simulink model "RL_sus_quarter_sim"  (R2025a)
settings: Solver=FixedStepAuto  StartTime=0.0  StopTime=20  FixedStep=0.001  RelTol=1e-3
model workspace (MAT data in the model file):
  G0 : Simulink.Parameter (value not decoded)
  Q_F : Simulink.Parameter (value not decoded)
  Q_dot_s : Simulink.Parameter (value not decoded)
  Q_dot_s_h : Simulink.Parameter (value not decoded)
  Q_dot_u : Simulink.Parameter (value not decoded)
  Q_flec : Simulink.Parameter (value not decoded)
  Q_flec_t : Simulink.Parameter (value not decoded)
  b_deflec : Simulink.Parameter (value not decoded)
  bump_height : Simulink.Parameter (value not decoded)
  bump_lenth : Simulink.Parameter (value not decoded)
  bump_start : Simulink.Parameter (value not decoded)
  f0 : Simulink.Parameter (value not decoded)
  kt : Simulink.Parameter (value not decoded)
  ms : Simulink.Parameter (value not decoded)
  n0 : Simulink.Parameter (value not decoded)
  n1 : Simulink.Parameter (value not decoded)
  omega_1 : Simulink.Parameter (value not decoded)
  omega_2 : Simulink.Parameter (value not decoded)
  omega_3 : Simulink.Parameter (value not decoded)
  omega_4 : Simulink.Parameter (value not decoded)
  ramp_height : Simulink.Parameter (value not decoded)
  ramp_lenth : Simulink.Parameter (value not decoded)
  ramp_start : Simulink.Parameter (value not decoded)
  sine_amp : Simulink.Parameter (value not decoded)
  sine_freq : Simulink.Parameter (value not decoded)
  u : Simulink.Parameter (value not decoded)
symbols that are objects in the model workspace (value not decoded): b_deflec, bump_height, bump_lenth, bump_start, f0, G0, kt, ms, n0, n1, omega_1, omega_2, omega_3, omega_4, Q_dot_s, Q_dot_s_h, Q_F, Q_flec, Q_flec_t, ramp_height, ramp_lenth, ramp_start, sine_amp, sine_freq
undefined symbols (not defined in the file): Ground, Hook, SH_ADD_new_as_as_xdef
libraries: fl_lib x250, nesl_utility x48, sharedTrackingLibrary x34, dspstat3 x18, simulink x3, deeplib x2, slpidlib x1
(part 6 of 12)

== system RL_sus_quarter_sim/Quarter_sys/Control/Y_1/IFEKF FDC/Subsystem ==
  v_s : Inport
  v_def : Inport  Port=2
  a_s : Inport  Port=3
  Abs : Abs  SaturateOnIntegerOverflow=off
  Constant : Constant  Value=1.4*2*pi
  Constant1 : Constant  Value=1.4*2*pi
  Constant2 : Constant  Value=3
  Constant8 : Constant  Value=0
  FS2 : Constant  Value=11
  FS3 : Constant  Value=15
  MATLAB Function : MATLAB Function  TreatAsAtomicUnit=on
  MATLAB Function1 : MATLAB Function  TreatAsAtomicUnit=on
  MATLAB Function2 : Subsystem  Variant=on  VariantControlMode=label  VariantControl=MATLAB Function1  LabelModeActiveChoice=adaptive IFEKF sdimple_3
  MATLAB Function3 : MATLAB Function  TreatAsAtomicUnit=on
  Multiport Switch : MultiPortSwitch  SaturateOnIntegerOverflow=off  InputSameDT=off
  Scope : Scope
      settings: ActiveDisplayYMinimum=8.52023  ActiveDisplayYMaximum=10.23596  DataLoggingVariableName=ScopeData4
  To Workspace : ToWorkspace  VariableName=est_omega  SampleTime=-1
  Zero-Order Hold : ZeroOrderHold  SampleTime=0.001
  FS_select : Outport
  wires:
  Constant8/1 -> MATLAB Function2/2(epsilon)
  Zero-Order Hold/1 -> MATLAB Function2/1(y)
  MATLAB Function2/6(omega) -> Abs/1
  Abs/1 -> MATLAB Function/1(u), MATLAB Function3/1(u), MATLAB Function1/1(u), To Workspace/1, Scope/1
  FS2/1 -> MATLAB Function/2(FS_2), MATLAB Function1/2(FS_2), MATLAB Function3/5(alpha2)
  MATLAB Function/1(y) -> Multiport Switch/2
  v_s/1 -> MATLAB Function1/3(vs), MATLAB Function3/2(vs), MATLAB Function/3(vs), Zero-Order Hold/1
  Constant/1 -> MATLAB Function/5(alpha), MATLAB Function1/5(alpha)
  v_def/1 -> MATLAB Function/4(vdef)
  MATLAB Function1/1(y) -> Multiport Switch/3
  Multiport Switch/1 -> FS_select/1
  a_s/1 -> MATLAB Function1/4(as), MATLAB Function3/3(as)
  MATLAB Function3/1(y) -> Multiport Switch/4
  Constant2/1 -> Multiport Switch/1
  Constant1/1 -> MATLAB Function3/4(alpha)
  FS3/1 -> MATLAB Function3/6(alpha3)

== system RL_sus_quarter_sim/Quarter_sys/Control/Y_1/IFEKF FDC/Subsystem1 ==
  v_def : Inport
  Gain : Gain  Gain=-1
  Lmbada_C : Constant  Value=1000
  Product1 : Product
  Out1 : Outport
  wires:
  Gain/1 -> Out1/1
  v_def/1 -> Product1/1
  Lmbada_C/1 -> Product1/2
  Product1/1 -> Gain/1

== system RL_sus_quarter_sim/Quarter_sys/Control/Y_1/IFEKF FDC/skyhook ==
  v_def : Inport
  v_s : Inport  Port=2
  Add : Sum
  Constant : Constant  Value=-1
  Constant1 : Constant
  Delta_C : Gain  Gain=500
  Gain : Gain  Gain=-1
  Lmbada_C : Constant  Value=1000
  Product : Product
  Product1 : Product
  Switch : Switch  Criteria=u2 > Threshold  SaturateOnIntegerOverflow=off  InputSameDT=off
  F_sus1 : Outport
  wires:
  v_def/1 -> Product/1, Product1/1
  Switch/1 -> Delta_C/1
  Add/1 -> Product1/2
  Constant/1 -> Switch/3
  Lmbada_C/1 -> Add/2
  v_s/1 -> Product/2
  Delta_C/1 -> Add/1
  Constant1/1 -> Switch/1
  Product1/1 -> Gain/1
  Product/1 -> Switch/2
  Gain/1 -> F_sus1/1

== system RL_sus_quarter_sim/Quarter_sys/Control/Y_1/IFEKF SHADD/ADD ==
  v_def : Inport
  a_s : Inport  Port=2
  Add : Sum
  Constant : Constant  Value=-1
  Constant1 : Constant
  Delta_C : Gain  Gain=500
  Gain1 : Gain  Gain=-1
  Lmbada_C : Constant  Value=1000
  Product : Product
  Product2 : Product
  Switch : Switch  Criteria=u2 > Threshold  SaturateOnIntegerOverflow=off  InputSameDT=off
  Out1 : Outport
  wires:
  Gain1/1 -> Out1/1
  Product/1 -> Switch/2
  Add/1 -> Product2/2
  Switch/1 -> Delta_C/1
  a_s/1 -> Product/2
  v_def/1 -> Product/1, Product2/1
  Product2/1 -> Gain1/1
  Constant/1 -> Switch/3
  Constant1/1 -> Switch/1
  Delta_C/1 -> Add/1
  Lmbada_C/1 -> Add/2

== system RL_sus_quarter_sim/Quarter_sys/Control/Y_1/IFEKF SHADD/Subsystem ==
  v_s : Inport
  Abs : Abs  SaturateOnIntegerOverflow=off
  Constant8 : Constant  Value=0
  FS1 : Constant  Value=1.4
  FS2 : Constant  Value=11
  FS3 : Constant  Value=19
  MATLAB Function : MATLAB Function  TreatAsAtomicUnit=on
  MATLAB Function2 : Subsystem  Variant=on  VariantControlMode=label  VariantControl=MATLAB Function1  LabelModeActiveChoice=adaptive IFEKF simple
  Scope : Scope
      settings: ActiveDisplayYMinimum=-3.68957  ActiveDisplayYMaximum=33.7061  DataLoggingVariableName=ScopeData4
  Zero-Order Hold : ZeroOrderHold  SampleTime=0.001
  FS_select : Outport
  wires:
  FS3/1 -> MATLAB Function/4(FS_3)
  MATLAB Function/1(y) -> FS_select/1
  FS2/1 -> MATLAB Function/3(FS_2)
  FS1/1 -> MATLAB Function/2(FS_1)
  Abs/1 -> MATLAB Function/1(u), Scope/1
  v_s/1 -> Zero-Order Hold/1
  MATLAB Function2/6(omega) -> Abs/1
  Zero-Order Hold/1 -> MATLAB Function2/1(y)
  Constant8/1 -> MATLAB Function2/2(epsilon)

== system RL_sus_quarter_sim/Quarter_sys/Control/Y_1/IFEKF SHADD/skyhook ==
  v_def : Inport
  v_s : Inport  Port=2
  Add : Sum
  Constant : Constant  Value=-1
  Constant1 : Constant
  Delta_C : Gain  Gain=500
  Gain : Gain  Gain=-1
  Lmbada_C : Constant  Value=1000
  Product : Product
  Product1 : Product
  Switch : Switch  Criteria=u2 > Threshold  SaturateOnIntegerOverflow=off  InputSameDT=off
  F_sus1 : Outport
  wires:
  Gain/1 -> F_sus1/1
  Product/1 -> Switch/2
  Product1/1 -> Gain/1
  Constant1/1 -> Switch/1
  Delta_C/1 -> Add/1
  v_s/1 -> Product/2
  Lmbada_C/1 -> Add/2
  Constant/1 -> Switch/3
  Add/1 -> Product1/2
  Switch/1 -> Delta_C/1
  v_def/1 -> Product1/1, Product/1

== system RL_sus_quarter_sim/Quarter_sys/Control/Y_1/IFEKF Select c/Subsystem ==
  In1 : Inport
  Abs : Abs  SaturateOnIntegerOverflow=off
  Constant8 : Constant  Value=0
  FS1 : Constant  Value=1.5
  FS2 : Constant  Value=10.2
  MATLAB Function : MATLAB Function  TreatAsAtomicUnit=on
  MATLAB Function2 : Subsystem  Variant=on  VariantControlMode=label  VariantControl=MATLAB Function1  LabelModeActiveChoice=adaptive IFEKF simple
  Scope : Scope
      settings: ActiveDisplayYMinimum=-3.69078  ActiveDisplayYMaximum=33.71699  DataLoggingVariableName=ScopeData4
  To Workspace : ToWorkspace  VariableName=freq_hat  SampleTime=-1
  Zero-Order Hold : ZeroOrderHold  SampleTime=0.001
  FS_select : Outport
  wires:
  Constant8/1 -> MATLAB Function2/2(epsilon)
  MATLAB Function2/5(y_residual) -> ?
  Zero-Order Hold/1 -> MATLAB Function2/1(y)
  MATLAB Function2/6(omega) -> To Workspace/1, Abs/1
  In1/1 -> Zero-Order Hold/1
  Abs/1 -> Scope/1, MATLAB Function/1(u)
  MATLAB Function2/1(x1hat) -> ?
  MATLAB Function2/3(debug) -> ?
  MATLAB Function2/4(xhat_pred) -> ?
  MATLAB Function2/2(P) -> ?
  FS1/1 -> MATLAB Function/2(FS_1)
  FS2/1 -> MATLAB Function/3(FS_2)
  MATLAB Function/1(y) -> FS_select/1

== system RL_sus_quarter_sim/Quarter_sys/Control/Y_1/IFEKF Select c/Subsystem2 ==
  sig select : Inport
  v_def : Inport  Port=2
  v_s : Inport  Port=3
  a_s : Inport  Port=4
  constant : Subsystem  VariantControl=constant
  semi ctr : Subsystem  VariantControl=semi active ctr
  F_damper : Outport

== system RL_sus_quarter_sim/Quarter_sys/Control/Y_1/IFEKF freq b/Subsystem ==
  v_s : Inport
  Abs : Abs  SaturateOnIntegerOverflow=off
  Constant8 : Constant  Value=0
  FS1 : Constant  Value=5
  FS2 : Constant  Value=11
  FS3 : Constant  Value=19
  MATLAB Function : MATLAB Function  TreatAsAtomicUnit=on
  MATLAB Function2 : Subsystem  Variant=on  VariantControlMode=label  VariantControl=MATLAB Function1  LabelModeActiveChoice=adaptive IFEKF simple
  Scope : Scope
      settings: ActiveDisplayYMinimum=-3.69075  ActiveDisplayYMaximum=33.71678  DataLoggingVariableName=ScopeData4
  Zero-Order Hold : ZeroOrderHold  SampleTime=0.001
  FS_select : Outport
  wires:
  Constant8/1 -> MATLAB Function2/2(epsilon)
  Zero-Order Hold/1 -> MATLAB Function2/1(y)
  MATLAB Function2/6(omega) -> Abs/1
  v_s/1 -> Zero-Order Hold/1
  Abs/1 -> Scope/1, MATLAB Function/1(u)
  FS1/1 -> MATLAB Function/2(FS_1)
  FS2/1 -> MATLAB Function/3(FS_2)
  MATLAB Function/1(y) -> FS_select/1
  FS3/1 -> MATLAB Function/4(FS_3)

== system RL_sus_quarter_sim/Quarter_sys/Control/Y_1/IFEKF freq b/large b ==
  a_def : Inport
  Gain : Gain  Gain=-1
  Product1 : Product
  b : Constant  Value=30
  F_sus1 : Outport
  wires:
  a_def/1 -> Product1/1
  Product1/1 -> Gain/1
  Gain/1 -> F_sus1/1
  b/1 -> Product1/2

== system RL_sus_quarter_sim/Quarter_sys/Control/Y_1/IFEKF freq b/mid b ==
  a_def : Inport
  Gain : Gain  Gain=-1
  Product1 : Product
  b : Constant  Value=10
  Out1 : Outport
  wires:
  Product1/1 -> Gain/1
  b/1 -> Product1/2
  a_def/1 -> Product1/1
  Gain/1 -> Out1/1

== system RL_sus_quarter_sim/Quarter_sys/Control/Y_1/IFEKF freq b/small  b ==
  a_def : Inport
  Gain : Gain  Gain=-1
  Product1 : Product
  b : Constant  Value=0
  Out1 : Outport
  wires:
  Gain/1 -> Out1/1
  a_def/1 -> Product1/1
  b/1 -> Product1/2
  Product1/1 -> Gain/1

== system RL_sus_quarter_sim/Quarter_sys/Control/Y_1/IFEKF freq bc/Subsystem ==
  v_s : Inport
  Abs : Abs  SaturateOnIntegerOverflow=off
  Constant8 : Constant  Value=0
  FS1 : Constant  Value=5
  FS2 : Constant  Value=11
  FS3 : Constant  Value=19
  MATLAB Function : MATLAB Function  TreatAsAtomicUnit=on
  MATLAB Function1 : MATLAB Function  TreatAsAtomicUnit=on
  MATLAB Function2 : Subsystem  Variant=on  VariantControlMode=label  VariantControl=MATLAB Function1  LabelModeActiveChoice=adaptive IFEKF simple
  Scope : Scope
      settings: ActiveDisplayYMinimum=-3.69075  ActiveDisplayYMaximum=33.71678  DataLoggingVariableName=ScopeData4
  Scope1 : Scope
      settings: ActiveDisplayYMinimum=0.875  ActiveDisplayYMaximum=2.125  DataLoggingVariableName=ScopeData9
  Scope2 : Scope
      settings: ActiveDisplayYMinimum=0.75  ActiveDisplayYMaximum=3.25  DataLoggingVariableName=ScopeData10
  Zero-Order Hold : ZeroOrderHold  SampleTime=0.001
  c FS1 : Constant  Value=1.5
  c FS2 : Constant  Value=11
  FS_select b : Outport
  FS_select c : Outport  Port=2
  wires:
  FS3/1 -> MATLAB Function/4(FS_3)
  MATLAB Function/1(y) -> Scope2/1, FS_select b/1
  FS2/1 -> MATLAB Function/3(FS_2)
  FS1/1 -> MATLAB Function/2(FS_1)
  Abs/1 -> MATLAB Function/1(u), Scope/1, MATLAB Function1/1(u)
  v_s/1 -> Zero-Order Hold/1
  MATLAB Function2/6(omega) -> Abs/1
  Zero-Order Hold/1 -> MATLAB Function2/1(y)
  Constant8/1 -> MATLAB Function2/2(epsilon)
  MATLAB Function1/1(y) -> Scope1/1, FS_select c/1
  c FS1/1 -> MATLAB Function1/2(FS_1)
  c FS2/1 -> MATLAB Function1/3(FS_2)

== system RL_sus_quarter_sim/Quarter_sys/Control/Y_1/IFEKF freq bc/large C ==
  v_def : Inport
  C : Constant  Value=2000
  Gain : Gain  Gain=-1
  Product1 : Product
  F_sus1 : Outport
  wires:
  v_def/1 -> Product1/1
  Product1/1 -> Gain/1
  Gain/1 -> F_sus1/1
  C/1 -> Product1/2

== system RL_sus_quarter_sim/Quarter_sys/Control/Y_1/IFEKF freq bc/large b ==
  a_def : Inport
  Gain : Gain  Gain=-1
  Product1 : Product
  b : Constant  Value=30
  F_sus1 : Outport
  wires:
  b/1 -> Product1/2
  Gain/1 -> F_sus1/1
  Product1/1 -> Gain/1
  a_def/1 -> Product1/1

== system RL_sus_quarter_sim/Quarter_sys/Control/Y_1/IFEKF freq bc/mid b ==
  a_def : Inport
  Gain : Gain  Gain=-1
  Product1 : Product
  b : Constant  Value=10
  Out1 : Outport
  wires:
  Gain/1 -> Out1/1
  a_def/1 -> Product1/1
  b/1 -> Product1/2
  Product1/1 -> Gain/1

== system RL_sus_quarter_sim/Quarter_sys/Control/Y_1/IFEKF freq bc/small  b ==
  a_def : Inport
  Gain : Gain  Gain=-1
  Product1 : Product
  b : Constant  Value=0
  Out1 : Outport
  wires:
  Product1/1 -> Gain/1
  b/1 -> Product1/2
  a_def/1 -> Product1/1
  Gain/1 -> Out1/1

== system RL_sus_quarter_sim/Quarter_sys/Control/Y_1/IFEKF freq bc/small C ==
  v_def : Inport
  C : Constant  Value=1000
  Gain : Gain  Gain=-1
  Product1 : Product
  Out1 : Outport
  wires:
  Gain/1 -> Out1/1
  v_def/1 -> Product1/1
  C/1 -> Product1/2
  Product1/1 -> Gain/1

== system RL_sus_quarter_sim/Quarter_sys/Control/Y_1/IFEKF freq bkkcc/Subsystem ==
  v_s : Inport
  Abs : Abs  SaturateOnIntegerOverflow=off
  Chart : Stateflow chart  TreatAsAtomicUnit=on  SystemSampleTime=0.001
  Chart1 : Stateflow chart  TreatAsAtomicUnit=on  SystemSampleTime=0.001
  Constant : Constant  Value=10000
  Constant1 : Constant  Value=10
  Constant2 : Constant  Value=1000
  Constant3 : Constant  Value=-500
  Constant4 : Constant  Value=-10000
  Constant5 : Constant  Value=30
  Constant6 : Constant  Value=3
  Constant8 : Constant  Value=0
  Demux : Demux  Outputs=2
  FS1 : Constant  Value=0.65
  FS2 : Constant  Value=4.5
  L1 : Subsystem
  L2 : Subsystem
  L3 : Subsystem
  MATLAB Function2 : Subsystem  Variant=on  VariantControlMode=label  VariantControl=MATLAB Function1  LabelModeActiveChoice=adaptive IFEKF simple
  Manual Switch : ManualSwitch
  Multiport Switch : MultiPortSwitch  Inputs=2  SaturateOnIntegerOverflow=off  InputSameDT=off
  Multiport Switch1 : MultiPortSwitch  Inputs=7  SaturateOnIntegerOverflow=off  InputSameDT=off
  Mux : Mux
  Mux1 : Mux  Inputs=2
  Mux2 : Mux  Inputs=2
  Scope : Scope
      settings: ActiveDisplayYMinimum=7.5  ActiveDisplayYMaximum=32.5
  Scope1 : Scope
      settings: ActiveDisplayYMinimum=-10696.7424  ActiveDisplayYMaximum=10249.86115  DataLoggingVariableName=ScopeData2
  Scope2 : Scope
      settings: ActiveDisplayYMinimum=0.875  ActiveDisplayYMaximum=2.125  DataLoggingVariableName=ScopeData3
  Zero-Order Hold : ZeroOrderHold  SampleTime=0.001
  passive : Subsystem
  Out1 : Outport
  wires:
  Constant8/1 -> MATLAB Function2/2(epsilon)
  Zero-Order Hold/1 -> MATLAB Function2/1(y)
  MATLAB Function2/6(omega) -> Abs/1
  v_s/1 -> Zero-Order Hold/1
  Abs/1 -> Chart/1(freq), Chart1/1(freq)
  FS1/1 -> Chart/2(FS1)
  FS2/1 -> Chart/3(FS2)
  Demux/1 -> Mux/1, Scope1/1  "k_a1"
  Constant3/1 -> Mux/2  "c_a1"
  Constant2/1 -> Mux/3  "c_a2"
  Demux/2 -> Scope/1, Mux/4  "b"
  Mux/1 -> ?
  Chart/1(level) -> Multiport Switch/1
  Multiport Switch/1 -> Demux/1
  Constant/1 -> Mux1/1  "ka1"
  Constant1/1 -> Mux1/2  "b"
  Mux1/1 -> Multiport Switch/2  "L1"
  Constant4/1 -> Mux2/1  "ka1"
  Constant5/1 -> Mux2/2  "b"
  Mux2/1 -> Multiport Switch/3  "L2"
  Chart1/1(level) -> Scope2/1, Manual Switch/1
  Multiport Switch1/1 -> Out1/1
  L1/1(Out1) -> Multiport Switch1/5, Multiport Switch1/8
  Manual Switch/1 -> Multiport Switch1/1
  Constant6/1 -> Manual Switch/2
  L3/1(Out1) -> Multiport Switch1/4, Multiport Switch1/7
  L2/1(Out1) -> Multiport Switch1/2, Multiport Switch1/3
  passive/1(Out1) -> Multiport Switch1/6

== system RL_sus_quarter_sim/Quarter_sys/Control/Y_1/IFEKF freq bkkcc/Subsystem1 ==
  input1 : Inport
  input0 : Inport  Port=2
  Ideal Force Sensor : fl_lib/Mechanical/Mechanical Sensors/Ideal Force Sensor
  Ideal Translational Velocity Source : fl_lib/Mechanical/Mechanical Sources/Ideal Translational Velocity Source
  Mechanical Translational Reference : fl_lib/Mechanical/Translational Elements/Mechanical Translational Reference
  Mechanical Translational Reference1 : fl_lib/Mechanical/Translational Elements/Mechanical Translational Reference
  PS-Simulink Converter : nesl_utility/PS-Simulink Converter  PhysicalDomain=network_engine_domain  SubClassName=ps_output  LeftPortType=input  RightPortType=output  PseudoPeriodic=off  Frequencies=[]  VectorFormat=inherit  Unit=inherit  AffineConversion=off
  Simulink-PS Converter : nesl_utility/Simulink-PS Converter  PhysicalDomain=network_engine_domain  SubClassName=ps_input  LeftPortType=input  RightPortType=output  PseudoPeriodic=off  Frequencies=[]  NoiseDistribution=none  NoiseParameters=[]  Unit=1  AffineConversion=off  FilteringAndDerivatives=provide  SimscapeFilterOrder=1  InputFilterTimeConstant=0.001  UdotUserProvided=1
  Solver Configuration : nesl_utility/Solver Configuration  PhysicalDomain=network_engine_domain  SubClassName=solver  LeftPortType=input  RightPortType=generic  Tones=[]  Harmonics=[]  SimulateNoise=off  Profile=off  UseLocalSampling=off  EnableSwitchedLinearOptims=on  FrequencyDomain=off  UseCCode=off  RelTol=0.001  AbsTol=0.001  MinStep=1e-09  ToWorkspace=off  RevertToSquareIcSolve=off  NumHomotopyIterations=100  PhasorMode=off  PhasorModeNumHarmonics=1  ConsistencySolver=NEWTON_XTOL_AFTER_FTOL  IndexReductionMethod=DerivativeReplacement  DoDC=off  ResidualTolerance=1e-09  ConsistencyTolSource=GLOBAL  ConsistencyAbsTol=0.001  ConsistencyRelTol=0.001  ConsistencyTolFactor=0.001  UseLocalSolver=off  LocalSolverChoice=NE_BACKWARD_EULER_ADVANCER  ResolveIndetEquations=on  FunctionEvalNumThread=1  LocalSolverSampleTime=0.001  DoFixedCost=off  MaxNonlinIter=3  MaxModeIter=2  ComputeImpulses=off  ImpulseIterations=2  LinearAlgebra=auto  LinearAlgebraNumThread=0  EquationFormulation=NE_TIME_EF  DelaysMemoryBudget=1024  AutomaticFiltering=on  FilteringTimeConstant=0.001  PartitionStorageMethod=AS_NEEDED  PartitionMemoryBudget=1024  PartitionMethod=ROBUST  MultibodyUseLocalSolver=off  MultibodyLocalSolverChoice=ODE1  MultibodyLocalSolverSampleTime=0.001
  Subsystem1 : Subsystem
  output : Outport
  wires:
  PS-Simulink Converter/1 -> output/1
  input0/1 -> Simulink-PS Converter/1
  input1/1 -> Simulink-PS Converter/2
  connections:
  Simulink-PS Converter/RConn1 -- Ideal Translational Velocity Source/RConn1
  Subsystem1/LConn1 -- Ideal Translational Velocity Source/RConn2
  Ideal Force Sensor/RConn1 -- Mechanical Translational Reference/LConn1
  Ideal Force Sensor/LConn1 -- Subsystem1/RConn1
  Mechanical Translational Reference1/LConn1 -- Solver Configuration/RConn1 -- Ideal Translational Velocity Source/LConn1
  PS-Simulink Converter/LConn1 -- Ideal Force Sensor/RConn2

== system RL_sus_quarter_sim/Quarter_sys/Control/Y_1/IFEKF freq bkkcc/bkkcc ==
  v_def : Inport
  x_def : Inport  Port=2
  a_def : Inport  Port=3
  param_ctr : Inport  Port=4
  Add : Sum  Inputs=+++
  Add1 : Sum
  Demux : Demux
  Divide : Product  Inputs=*/
  Gain{,1..3} (4 alike) : Gain  Gain=-1
  Integrator : Integrator
  Product{,1..3} (4 alike) : Product
  F_bkkcc : Outport
  wires:
  x_def/1 -> Product/2
  Demux/1 -> Gain/1  "k_a1"
  Product/1 -> Add/1
  Demux/2 -> Gain1/1  "c_a1"
  Product1/1 -> Add/2
  Add/1 -> F_bkkcc/1
  Demux/3 -> Product3/1, Gain2/1  "c_a2"
  Demux/4 -> Gain3/1  "b"
  Product2/1 -> Add/3
  Gain/1 -> Product/1
  Gain1/1 -> Product1/1
  Gain2/1 -> Product2/1
  Gain3/1 -> Divide/2
  param_ctr/1 -> Demux/1
  Add1/1 -> Integrator/1  "a1"
  Divide/1 -> Add1/1
  a_def/1 -> Add1/2
  v_def/1 -> Product1/2
  Integrator/1 -> Product2/2, Product3/2  "v1"
  Product3/1 -> Divide/1

== system RL_sus_quarter_sim/Quarter_sys/Control/Y_1/IFEKF freq c/Large C ==
  v_def : Inport
  Gain : Gain  Gain=-1
  Lmbada_C : Constant  Value=1500
  Product1 : Product
  Out1 : Outport
  wires:
  Gain/1 -> Out1/1
  v_def/1 -> Product1/1
  Lmbada_C/1 -> Product1/2
  Product1/1 -> Gain/1

== system RL_sus_quarter_sim/Quarter_sys/Control/Y_1/IFEKF freq c/Mid C ==
  v_def : Inport
  Gain : Gain  Gain=-1
  Lmbada_C : Constant  Value=1000
  Product1 : Product
  Out1 : Outport
  wires:
  Gain/1 -> Out1/1
  v_def/1 -> Product1/1
  Lmbada_C/1 -> Product1/2
  Product1/1 -> Gain/1

== system RL_sus_quarter_sim/Quarter_sys/Control/Y_1/IFEKF freq c/Small C ==
  v_def : Inport
  Gain : Gain  Gain=-1
  Lmbada_C : Constant  Value=500
  Product1 : Product
  Out1 : Outport
  wires:
  Product1/1 -> Gain/1
  Lmbada_C/1 -> Product1/2
  v_def/1 -> Product1/1
  Gain/1 -> Out1/1

== system RL_sus_quarter_sim/Quarter_sys/Control/Y_1/IFEKF freq c/Subsystem ==
  v_s : Inport
  Abs : Abs  SaturateOnIntegerOverflow=off
  Constant8 : Constant  Value=0
  FF-1 : Constant  Value=11.3
  FL-1 : Constant  Value=1.33
  FL-2 : Constant  Value=12.4
  MATLAB Function : MATLAB Function  TreatAsAtomicUnit=on
  MATLAB Function2 : Subsystem  Variant=on  VariantControlMode=label  VariantControl=MATLAB Function1  LabelModeActiveChoice=adaptive IFEKF simple
  Scope : Scope
      settings: ActiveDisplayYMinimum=-0.50296  ActiveDisplayYMaximum=5.02664  DataLoggingVariableName=ScopeData4
  Zero-Order Hold : ZeroOrderHold  SampleTime=0.001
  FS_select : Outport
  wires:
  Constant8/1 -> MATLAB Function2/2(epsilon)
  Zero-Order Hold/1 -> MATLAB Function2/1(y)
  MATLAB Function2/6(omega) -> Abs/1
  v_s/1 -> Zero-Order Hold/1
  Abs/1 -> Scope/1, MATLAB Function/1(u)
  FL-1/1 -> MATLAB Function/2(FS_1)
  FF-1/1 -> MATLAB Function/3(FS_2)
  MATLAB Function/1(y) -> FS_select/1
  FL-2/1 -> MATLAB Function/4(FS_3)

== system RL_sus_quarter_sim/Quarter_sys/Control/Y_1/PA bk/Subsystem ==
  input0 : Inport
  input1 : Inport  Port=2
  Ideal Force Sensor : fl_lib/Mechanical/Mechanical Sensors/Ideal Force Sensor
  Ideal Translational Velocity Source : fl_lib/Mechanical/Mechanical Sources/Ideal Translational Velocity Source
  Mechanical Translational Reference : fl_lib/Mechanical/Translational Elements/Mechanical Translational Reference
  Mechanical Translational Reference1 : fl_lib/Mechanical/Translational Elements/Mechanical Translational Reference
  PS-Simulink Converter : nesl_utility/PS-Simulink Converter  PhysicalDomain=network_engine_domain  SubClassName=ps_output  LeftPortType=input  RightPortType=output  PseudoPeriodic=off  Frequencies=[]  VectorFormat=inherit  Unit=inherit  AffineConversion=off
  Simulink-PS Converter : nesl_utility/Simulink-PS Converter  PhysicalDomain=network_engine_domain  SubClassName=ps_input  LeftPortType=input  RightPortType=output  PseudoPeriodic=off  Frequencies=[]  NoiseDistribution=none  NoiseParameters=[]  Unit=1  AffineConversion=off  FilteringAndDerivatives=provide  SimscapeFilterOrder=1  InputFilterTimeConstant=0.001  UdotUserProvided=1
  Solver Configuration : nesl_utility/Solver Configuration  PhysicalDomain=network_engine_domain  SubClassName=solver  LeftPortType=input  RightPortType=generic  Tones=[]  Harmonics=[]  SimulateNoise=off  Profile=off  UseLocalSampling=off  EnableSwitchedLinearOptims=on  FrequencyDomain=off  UseCCode=off  RelTol=0.001  AbsTol=0.001  MinStep=1e-09  ToWorkspace=off  RevertToSquareIcSolve=off  NumHomotopyIterations=100  PhasorMode=off  PhasorModeNumHarmonics=1  ConsistencySolver=NEWTON_XTOL_AFTER_FTOL  IndexReductionMethod=DerivativeReplacement  DoDC=off  ResidualTolerance=1e-09  ConsistencyTolSource=GLOBAL  ConsistencyAbsTol=0.001  ConsistencyRelTol=0.001  ConsistencyTolFactor=0.001  UseLocalSolver=off  LocalSolverChoice=NE_BACKWARD_EULER_ADVANCER  ResolveIndetEquations=on  FunctionEvalNumThread=1  LocalSolverSampleTime=0.001  DoFixedCost=off  MaxNonlinIter=3  MaxModeIter=2  ComputeImpulses=off  ImpulseIterations=2  LinearAlgebra=auto  LinearAlgebraNumThread=0  EquationFormulation=NE_TIME_EF  DelaysMemoryBudget=1024  AutomaticFiltering=on  FilteringTimeConstant=0.001  PartitionStorageMethod=AS_NEEDED  PartitionMemoryBudget=1024  PartitionMethod=ROBUST  MultibodyUseLocalSolver=off  MultibodyLocalSolverChoice=ODE1  MultibodyLocalSolverSampleTime=0.001
  Subsystem1 : Subsystem
  output : Outport
  wires:
  PS-Simulink Converter/1 -> output/1
  input0/1 -> Simulink-PS Converter/1
  input1/1 -> Simulink-PS Converter/2
  connections:
  Simulink-PS Converter/RConn1 -- Ideal Translational Velocity Source/RConn1
  Subsystem1/LConn1 -- Ideal Translational Velocity Source/RConn2
  Ideal Force Sensor/RConn1 -- Mechanical Translational Reference/LConn1
  Ideal Force Sensor/LConn1 -- Subsystem1/RConn1
  Solver Configuration/RConn1 -- Ideal Translational Velocity Source/LConn1 -- Mechanical Translational Reference1/LConn1
  PS-Simulink Converter/LConn1 -- Ideal Force Sensor/RConn2

== system RL_sus_quarter_sim/Quarter_sys/Control/Y_1/PA bkc/Subsystem ==
  input0 : Inport
  input1 : Inport  Port=2
  Ideal Force Sensor : fl_lib/Mechanical/Mechanical Sensors/Ideal Force Sensor
  Ideal Translational Velocity Source : fl_lib/Mechanical/Mechanical Sources/Ideal Translational Velocity Source
  Mechanical Translational Reference : fl_lib/Mechanical/Translational Elements/Mechanical Translational Reference
  Mechanical Translational Reference1 : fl_lib/Mechanical/Translational Elements/Mechanical Translational Reference
  PS-Simulink Converter : nesl_utility/PS-Simulink Converter  PhysicalDomain=network_engine_domain  SubClassName=ps_output  LeftPortType=input  RightPortType=output  PseudoPeriodic=off  Frequencies=[]  VectorFormat=inherit  Unit=inherit  AffineConversion=off
  Simulink-PS Converter : nesl_utility/Simulink-PS Converter  PhysicalDomain=network_engine_domain  SubClassName=ps_input  LeftPortType=input  RightPortType=output  PseudoPeriodic=off  Frequencies=[]  NoiseDistribution=none  NoiseParameters=[]  Unit=1  AffineConversion=off  FilteringAndDerivatives=provide  SimscapeFilterOrder=1  InputFilterTimeConstant=0.001  UdotUserProvided=1
  Solver Configuration : nesl_utility/Solver Configuration  PhysicalDomain=network_engine_domain  SubClassName=solver  LeftPortType=input  RightPortType=generic  Tones=[]  Harmonics=[]  SimulateNoise=off  Profile=off  UseLocalSampling=off  EnableSwitchedLinearOptims=on  FrequencyDomain=off  UseCCode=off  RelTol=0.001  AbsTol=0.001  MinStep=1e-09  ToWorkspace=off  RevertToSquareIcSolve=off  NumHomotopyIterations=100  PhasorMode=off  PhasorModeNumHarmonics=1  ConsistencySolver=NEWTON_XTOL_AFTER_FTOL  IndexReductionMethod=DerivativeReplacement  DoDC=off  ResidualTolerance=1e-09  ConsistencyTolSource=GLOBAL  ConsistencyAbsTol=0.001  ConsistencyRelTol=0.001  ConsistencyTolFactor=0.001  UseLocalSolver=off  LocalSolverChoice=NE_BACKWARD_EULER_ADVANCER  ResolveIndetEquations=on  FunctionEvalNumThread=1  LocalSolverSampleTime=0.001  DoFixedCost=off  MaxNonlinIter=3  MaxModeIter=2  ComputeImpulses=off  ImpulseIterations=2  LinearAlgebra=auto  LinearAlgebraNumThread=0  EquationFormulation=NE_TIME_EF  DelaysMemoryBudget=1024  AutomaticFiltering=on  FilteringTimeConstant=0.001  PartitionStorageMethod=AS_NEEDED  PartitionMemoryBudget=1024  PartitionMethod=ROBUST  MultibodyUseLocalSolver=off  MultibodyLocalSolverChoice=ODE1  MultibodyLocalSolverSampleTime=0.001
  Subsystem1 : Subsystem
  output : Outport
  wires:
  input1/1 -> Simulink-PS Converter/2
  input0/1 -> Simulink-PS Converter/1
  PS-Simulink Converter/1 -> output/1
  connections:
  PS-Simulink Converter/LConn1 -- Ideal Force Sensor/RConn2
  Ideal Translational Velocity Source/LConn1 -- Solver Configuration/RConn1 -- Mechanical Translational Reference1/LConn1
  Ideal Force Sensor/LConn1 -- Subsystem1/RConn1
  Ideal Force Sensor/RConn1 -- Mechanical Translational Reference/LConn1
  Subsystem1/LConn1 -- Ideal Translational Velocity Source/RConn2
  Simulink-PS Converter/RConn1 -- Ideal Translational Velocity Source/RConn1

== system RL_sus_quarter_sim/Quarter_sys/Control/Y_1/PA bkkcc/Subsystem ==
  input0 : Inport
  input1 : Inport  Port=2
  Ideal Force Sensor : fl_lib/Mechanical/Mechanical Sensors/Ideal Force Sensor
  Ideal Translational Velocity Source : fl_lib/Mechanical/Mechanical Sources/Ideal Translational Velocity Source
  Mechanical Translational Reference : fl_lib/Mechanical/Translational Elements/Mechanical Translational Reference
  Mechanical Translational Reference1 : fl_lib/Mechanical/Translational Elements/Mechanical Translational Reference
  PS-Simulink Converter : nesl_utility/PS-Simulink Converter  PhysicalDomain=network_engine_domain  SubClassName=ps_output  LeftPortType=input  RightPortType=output  PseudoPeriodic=off  Frequencies=[]  VectorFormat=inherit  Unit=inherit  AffineConversion=off
  Simulink-PS Converter : nesl_utility/Simulink-PS Converter  PhysicalDomain=network_engine_domain  SubClassName=ps_input  LeftPortType=input  RightPortType=output  PseudoPeriodic=off  Frequencies=[]  NoiseDistribution=none  NoiseParameters=[]  Unit=1  AffineConversion=off  FilteringAndDerivatives=provide  SimscapeFilterOrder=1  InputFilterTimeConstant=0.001  UdotUserProvided=1
  Solver Configuration : nesl_utility/Solver Configuration  PhysicalDomain=network_engine_domain  SubClassName=solver  LeftPortType=input  RightPortType=generic  Tones=[]  Harmonics=[]  SimulateNoise=off  Profile=off  UseLocalSampling=off  EnableSwitchedLinearOptims=on  FrequencyDomain=off  UseCCode=off  RelTol=0.001  AbsTol=0.001  MinStep=1e-09  ToWorkspace=off  RevertToSquareIcSolve=off  NumHomotopyIterations=100  PhasorMode=off  PhasorModeNumHarmonics=1  ConsistencySolver=NEWTON_XTOL_AFTER_FTOL  IndexReductionMethod=DerivativeReplacement  DoDC=off  ResidualTolerance=1e-09  ConsistencyTolSource=GLOBAL  ConsistencyAbsTol=0.001  ConsistencyRelTol=0.001  ConsistencyTolFactor=0.001  UseLocalSolver=off  LocalSolverChoice=NE_BACKWARD_EULER_ADVANCER  ResolveIndetEquations=on  FunctionEvalNumThread=1  LocalSolverSampleTime=0.001  DoFixedCost=off  MaxNonlinIter=3  MaxModeIter=2  ComputeImpulses=off  ImpulseIterations=2  LinearAlgebra=auto  LinearAlgebraNumThread=0  EquationFormulation=NE_TIME_EF  DelaysMemoryBudget=1024  AutomaticFiltering=on  FilteringTimeConstant=0.001  PartitionStorageMethod=AS_NEEDED  PartitionMemoryBudget=1024  PartitionMethod=ROBUST  MultibodyUseLocalSolver=off  MultibodyLocalSolverChoice=ODE1  MultibodyLocalSolverSampleTime=0.001
  Subsystem1 : Subsystem
  output : Outport
  wires:
  PS-Simulink Converter/1 -> output/1
  input0/1 -> Simulink-PS Converter/1
  input1/1 -> Simulink-PS Converter/2
  connections:
  Simulink-PS Converter/RConn1 -- Ideal Translational Velocity Source/RConn1
  Subsystem1/LConn1 -- Ideal Translational Velocity Source/RConn2
  Ideal Force Sensor/RConn1 -- Mechanical Translational Reference/LConn1
  Ideal Force Sensor/LConn1 -- Subsystem1/RConn1
  Mechanical Translational Reference1/LConn1 -- Solver Configuration/RConn1 -- Ideal Translational Velocity Source/LConn1
  PS-Simulink Converter/LConn1 -- Ideal Force Sensor/RConn2

== system RL_sus_quarter_sim/Quarter_sys/Control/Y_1/P_0/Subsystem ==
  p0_k2 : Subsystem  VariantControl=p0_k2
  p0_k3 : Subsystem  VariantControl=p0_k3
  p0_k4 : Subsystem  VariantControl=p0_k4
  p0_k6 : Subsystem  VariantControl=p0_k6
  passive : Subsystem  VariantControl=passive
  Conn1 : PMIOPort  Side=Right
  Conn2 : PMIOPort  Port=2  Side=Left

== system RL_sus_quarter_sim/Quarter_sys/Control/Y_1/P_1/Subsystem ==
  p1_k1 : Subsystem  VariantControl=p1_k1
  p1_k2 : Subsystem  VariantControl=p1_k2
  p1_k3 : Subsystem  VariantControl=p1_k3
  p1_k5 : Subsystem  VariantControl=p1_k5
  passive : Subsystem  VariantControl=passive
  Conn1 : PMIOPort  Side=Right
  Conn2 : PMIOPort  Port=2  Side=Left

== system RL_sus_quarter_sim/Quarter_sys/Control/Y_1/P_test/Subsystem ==
  p1_k1 : Subsystem  VariantControl=p1_k1
  p1_k2 : Subsystem  VariantControl=p1_k2
  p1_k3 : Subsystem  VariantControl=p1_k3
  p1_k5 : Subsystem  VariantControl=p1_k5
  passive : Subsystem  VariantControl=passive
  Conn1 : PMIOPort  Side=Right
  Conn2 : PMIOPort  Port=2  Side=Left

== system RL_sus_quarter_sim/Quarter_sys/Control/Y_1/Pabbkk/Subsystem ==
  p1_k1 : Subsystem  VariantControl=p1_k1
  p1_k2 : Subsystem  VariantControl=p1_k2
  p1_k3 : Subsystem  VariantControl=p1_k3
  p1_k5 : Subsystem  VariantControl=p1_k5
  passive : Subsystem  VariantControl=passive
  Conn1 : PMIOPort  Side=Right
  Conn2 : PMIOPort  Port=2  Side=Left

== system RL_sus_quarter_sim/Quarter_sys/Control/Y_1/SH_ADD_modify/ADD1 ==
  v_def : Inport
  a_s : Inport  Port=2
  Constant2 : Constant  Value=500
  Constant3 : Constant  Value=1500
  Product : Product
  Switch : Switch  Criteria=u2 > Threshold  SaturateOnIntegerOverflow=off  InputSameDT=off
  F_sus1 : Outport
  wires:
  Product/1 -> Switch/2
  Constant2/1 -> Switch/3
  a_s/1 -> Product/2
  v_def/1 -> Product/1
  Constant3/1 -> Switch/1
  Switch/1 -> F_sus1/1

== system RL_sus_quarter_sim/Quarter_sys/Control/Y_1/SH_ADD_modify/Modify_SHADD ==
  v_def : Inport
  a_s : Inport  Port=2
  v_s : Inport  Port=3
  Multiport Switch1 : MultiPortSwitch  Inputs=2  SaturateOnIntegerOverflow=off  InputSameDT=off
  currency_ctr1 : Outport
  wires:
  Multiport Switch1/1 -> currency_ctr1/1

== system RL_sus_quarter_sim/Quarter_sys/Control/Y_1/SH_ADD_modify/SH1 ==
  v_def : Inport
  v_s : Inport  Port=2
  Constant2 : Constant  Value=500
  Constant3 : Constant  Value=1500
  Product : Product
  Switch : Switch  Criteria=u2 > Threshold  SaturateOnIntegerOverflow=off  InputSameDT=off
  Out1 : Outport
  wires:
  Product/1 -> Switch/2
  Constant3/1 -> Switch/1
  Constant2/1 -> Switch/3
  v_def/1 -> Product/1
  v_s/1 -> Product/2
  Switch/1 -> Out1/1

== system RL_sus_quarter_sim/Quarter_sys/Control/Y_1/SH_ADD_new_FS/Modify_SHADD ==
  v_def : Inport
  a_s : Inport  Port=2
  v_s : Inport  Port=3
  ADD1 : Subsystem
  Gain1 : Gain  Gain=2*pi
  MATLAB Function : MATLAB Function  TreatAsAtomicUnit=on
  Multiport Switch1 : MultiPortSwitch  Inputs=2  SaturateOnIntegerOverflow=off  InputSameDT=off
  SH1 : Subsystem
  alpha1 : Constant  Value=1.41
  cs : Constant  Value=1000
  ks : Constant  Value=20000
  ms : Constant  Value=400
  currency_ctr1 : Outport
  wires:
  MATLAB Function/1(y) -> Multiport Switch1/1
  a_s/1 -> ADD1/2(a_s)
  v_def/1 -> ADD1/1(v_def), MATLAB Function/2(vdef), SH1/1(v_def)
  Multiport Switch1/1 -> currency_ctr1/1
  v_s/1 -> MATLAB Function/1(vs), SH1/2(v_s)
  SH1/1(Out1) -> Multiport Switch1/2
  ADD1/1(F_sus1) -> Multiport Switch1/3
  alpha1/1 -> Gain1/1
  cs/1 -> MATLAB Function/4(cs)
  ks/1 -> MATLAB Function/5(ks)
  ms/1 -> MATLAB Function/6(ms)
  Gain1/1 -> MATLAB Function/3(alpha)

== system RL_sus_quarter_sim/Quarter_sys/Control/Y_1/SH_ADD_new_as_as_xdef^2/2nd_FS_adef_vs ==
  as : Inport
  xdef : Inport  Port=2
  2nd_FS : Sum  Inputs=-+
  Constant4 : Constant  Value=20000
  Constant5 : Constant  Value=400
  Constant6 : Constant  Value=1000
  MATLAB Function1 : MATLAB Function  TreatAsAtomicUnit=on
  Product : Product
  Scope : Scope  NumInputPorts=2
      settings: ActiveDisplayYMinimum=-153.06283  ActiveDisplayYMaximum=2530.22116  DataLoggingVariableName=ScopeData20
  Scope1 : Scope
      settings: ActiveDisplayYMinimum=-4.46239  ActiveDisplayYMaximum=40.1615  DataLoggingVariableName=ScopeData22
  Scope2 : Scope
      settings: ActiveDisplayYMinimum=-8.251717601977E+7  ActiveDisplayYMaximum=7.4265458417791E+8  DataLoggingVariableName=ScopeData23
  Scope3 : Scope
      settings: ActiveDisplayYMinimum=-101.89927  ActiveDisplayYMaximum=101.85233  DataLoggingVariableName=ScopeData24
  Square : Math  Operator=square
  Square1 : Math  Operator=square
  alpha2 : Constant  Value=2*2*pi
  FS2 : Outport
  wires:
  alpha2/1 -> Square/1, MATLAB Function1/3(alpha)
  Square/1 -> Product/1
  Constant5/1 -> MATLAB Function1/5(ms)
  2nd_FS/1 -> FS2/1
  MATLAB Function1/1(y) -> 2nd_FS/1, Scope2/1, Scope/1
  Constant6/1 -> MATLAB Function1/6(cs)
  Constant4/1 -> MATLAB Function1/4(ks)
  Product/1 -> Scope/2, 2nd_FS/2, Scope1/1
  as/1 -> Square1/1, MATLAB Function1/1(as), Scope3/1
  Square1/1 -> Product/2
  xdef/1 -> MATLAB Function1/2(xdef)

== system RL_sus_quarter_sim/Quarter_sys/Control/Y_1/SH_ADD_new_as_as_xdef^2/ADD ==
  x_def : Inport
  v_def : Inport  Port=2
  a_s : Inport  Port=3
  Add : Sum
  Add1 : Sum
  Constant7 : Constant  Value=-1
  Constant8 : Constant
  Delta_C : Gain  Gain=500
  Gain : Gain  Gain=-1
  Lmbada_C : Constant  Value=1000
  Product : Product
  Product1 : Product
  Switch : Switch  Criteria=u2 > Threshold  SaturateOnIntegerOverflow=off  InputSameDT=off
  ks : Gain  Gain=-20000
  F_sus1 : Outport
  wires:
  Gain/1 -> Add1/1
  Delta_C/1 -> Add/1
  Constant8/1 -> Switch/1
  Add/1 -> Product1/2
  Add1/1 -> F_sus1/1
  x_def/1 -> ks/1
  Lmbada_C/1 -> Add/2
  Product/1 -> Switch/2
  Product1/1 -> Gain/1
  Switch/1 -> Delta_C/1
  Constant7/1 -> Switch/3
  a_s/1 -> Product/2
  v_def/1 -> Product/1, Product1/1
  ks/1 -> Add1/2

== system RL_sus_quarter_sim/Quarter_sys/Control/Y_1/SH_ADD_new_as_as_xdef^2/SH ==
  v_def : Inport
  v_s : Inport  Port=2
  x_def : Inport  Port=3
  Add : Sum
  Add1 : Sum
  Constant : Constant  Value=-1
  Constant1 : Constant
  Delta_C : Gain  Gain=500
  Gain : Gain  Gain=-1
  Lmbada_C : Constant  Value=1000
  Product : Product
  Product1 : Product
  Switch : Switch  Criteria=u2 > Threshold  SaturateOnIntegerOverflow=off  InputSameDT=off
  ks : Gain  Gain=-20000
  Out1 : Outport
  wires:
  Product/1 -> Switch/2
  Delta_C/1 -> Add/1
  Lmbada_C/1 -> Add/2
  ks/1 -> Add1/2
  x_def/1 -> ks/1
  Constant1/1 -> Switch/1
  Product1/1 -> Gain/1
  Add/1 -> Product1/2
  Gain/1 -> Add1/1
  Constant/1 -> Switch/3
  v_def/1 -> Product1/1, Product/1
  Switch/1 -> Delta_C/1
  v_s/1 -> Product/2
  Add1/1 -> Out1/1

== system RL_sus_quarter_sim/Quarter_sys/Control/Y_1/SH_ADD_new_as_au_xdef_vdef/2nd_FS_adef_vs ==
  as : Inport
  xdef : Inport  Port=2
  vdef : Inport  Port=3
  au : Inport  Port=4
  2nd_FS : Sum  Inputs=-+
  Constant4 : Constant  Value=20000
  Constant5 : Constant  Value=400
  Constant6 : Constant  Value=1000
  MATLAB Function1 : MATLAB Function  TreatAsAtomicUnit=on
  Product : Product  Inputs=3
  Scope : Scope  NumInputPorts=2
      settings: ActiveDisplayYMinimum=-242980.23845  ActiveDisplayYMaximum=1.54576790077E+6  DataLoggingVariableName=ScopeData20
  Scope1 : Scope
      settings: ActiveDisplayYMinimum=-4.46239  ActiveDisplayYMaximum=40.1615  DataLoggingVariableName=ScopeData22
  Scope2 : Scope
      settings: ActiveDisplayYMinimum=-945.42406  ActiveDisplayYMaximum=8508.81651  DataLoggingVariableName=ScopeData23
  Scope3 : Scope
      settings: ActiveDisplayYMinimum=-101.89927  ActiveDisplayYMaximum=101.85233  DataLoggingVariableName=ScopeData24
  Square : Math  Operator=square
  Square1 : Math  Operator=square
  Square2 : Math  Operator=square
  alpha2 : Constant  Value=5*2*pi
  FS2 : Outport
  wires:
  xdef/1 -> MATLAB Function1/1(xdef)
  Square1/1 -> Product/2
  as/1 -> Scope3/1, Square1/1
  Product/1 -> 2nd_FS/2, Scope/2, Scope1/1
  Constant4/1 -> MATLAB Function1/4(ks)
  Constant6/1 -> MATLAB Function1/6(cs)
  MATLAB Function1/1(y) -> Scope/1, Scope2/1, 2nd_FS/1
  2nd_FS/1 -> FS2/1
  Constant5/1 -> MATLAB Function1/5(ms)
  Square/1 -> Product/1
  alpha2/1 -> MATLAB Function1/3(alpha), Square/1
  vdef/1 -> MATLAB Function1/2(vdef)
  au/1 -> Square2/1
  Square2/1 -> Product/3

== system RL_sus_quarter_sim/Quarter_sys/Control/Y_1/SH_ADD_new_as_au_xdef_vdef/ADD ==
  x_def : Inport
  v_def : Inport  Port=2
  a_s : Inport  Port=3
  Add : Sum
  Add1 : Sum
  Constant7 : Constant  Value=-1
  Constant8 : Constant
  Delta_C : Gain  Gain=500
  Gain : Gain  Gain=-1
  Lmbada_C : Constant  Value=1000
  Product : Product
  Product1 : Product
  Switch : Switch  Criteria=u2 > Threshold  SaturateOnIntegerOverflow=off  InputSameDT=off
  ks : Gain  Gain=-20000
  F_sus1 : Outport
  wires:
  ks/1 -> Add1/2
  v_def/1 -> Product1/1, Product/1
  a_s/1 -> Product/2
  Constant7/1 -> Switch/3
  Switch/1 -> Delta_C/1
  Product1/1 -> Gain/1
  Product/1 -> Switch/2
  Lmbada_C/1 -> Add/2
  x_def/1 -> ks/1
  Add1/1 -> F_sus1/1
  Add/1 -> Product1/2
  Constant8/1 -> Switch/1
  Delta_C/1 -> Add/1
  Gain/1 -> Add1/1

== system RL_sus_quarter_sim/Quarter_sys/Control/Y_1/SH_ADD_new_as_au_xdef_vdef/SH ==
  v_def : Inport
  v_s : Inport  Port=2
  x_def : Inport  Port=3
  Add : Sum
  Add1 : Sum
  Constant : Constant  Value=-1
  Constant1 : Constant
  Delta_C : Gain  Gain=500
  Gain : Gain  Gain=-1
  Lmbada_C : Constant  Value=1000
  Product : Product
  Product1 : Product
  Switch : Switch  Criteria=u2 > Threshold  SaturateOnIntegerOverflow=off  InputSameDT=off
  ks : Gain  Gain=-20000
  Out1 : Outport
  wires:
  Add1/1 -> Out1/1
  v_s/1 -> Product/2
  Switch/1 -> Delta_C/1
  v_def/1 -> Product/1, Product1/1
  Constant/1 -> Switch/3
  Gain/1 -> Add1/1
  Add/1 -> Product1/2
  Product1/1 -> Gain/1
  Constant1/1 -> Switch/1
  x_def/1 -> ks/1
  ks/1 -> Add1/2
  Lmbada_C/1 -> Add/2
  Delta_C/1 -> Add/1
  Product/1 -> Switch/2

== system RL_sus_quarter_sim/Quarter_sys/Control/Y_1/SH_ADD_new_au_vs/2nd_FS ==
  vs : Inport
  au : Inport  Port=2
  2nd_FS : Sum  Inputs=+-
  Constant4 : Constant  Value=20000
  Constant5 : Constant  Value=400
  Constant6 : Constant  Value=1000
  MATLAB Function1 : MATLAB Function  TreatAsAtomicUnit=on
  Product : Product
  Square : Math  Operator=square
  Square1 : Math  Operator=square
  alpha2 : Constant  Value=2*2*pi
  FS2 : Outport
  wires:
  alpha2/1 -> Square/1, MATLAB Function1/2(alpha)
  Square/1 -> Product/1
  Constant5/1 -> MATLAB Function1/4(ms)
  2nd_FS/1 -> FS2/1
  MATLAB Function1/1(y) -> 2nd_FS/1
  Constant6/1 -> MATLAB Function1/5(cs)
  Constant4/1 -> MATLAB Function1/3(ks)
  Product/1 -> 2nd_FS/2
  au/1 -> MATLAB Function1/1(au)
  vs/1 -> Square1/1
  Square1/1 -> Product/2

== system RL_sus_quarter_sim/Quarter_sys/Control/Y_1/SH_ADD_new_au_vs/ADD ==
  x_def : Inport
  v_def : Inport  Port=2
  a_s : Inport  Port=3
  Add : Sum
  Add1 : Sum
  Constant7 : Constant  Value=-1
  Constant8 : Constant
  Delta_C : Gain  Gain=500
  Gain : Gain  Gain=-1
  Lmbada_C : Constant  Value=1000
  Product : Product
  Product1 : Product
  Switch : Switch  Criteria=u2 > Threshold  SaturateOnIntegerOverflow=off  InputSameDT=off
  ks : Gain  Gain=-20000
  F_sus1 : Outport
  wires:
  Gain/1 -> Add1/1
  Delta_C/1 -> Add/1
  Constant8/1 -> Switch/1
  Add/1 -> Product1/2
  Add1/1 -> F_sus1/1
  x_def/1 -> ks/1
  Lmbada_C/1 -> Add/2
  Product/1 -> Switch/2
  Product1/1 -> Gain/1
  Switch/1 -> Delta_C/1
  Constant7/1 -> Switch/3
  a_s/1 -> Product/2
  v_def/1 -> Product/1, Product1/1
  ks/1 -> Add1/2

== system RL_sus_quarter_sim/Quarter_sys/Control/Y_1/SH_ADD_new_au_vs/SH ==
  v_def : Inport
  v_s : Inport  Port=2
  x_def : Inport  Port=3
  Add : Sum
  Add1 : Sum
  Constant : Constant  Value=-1
  Constant1 : Constant
  Delta_C : Gain  Gain=500
  Gain : Gain  Gain=-1
  Lmbada_C : Constant  Value=1000
  Product : Product
  Product1 : Product
  Switch : Switch  Criteria=u2 > Threshold  SaturateOnIntegerOverflow=off  InputSameDT=off
  ks : Gain  Gain=-20000
  Out1 : Outport
  wires:
  Product/1 -> Switch/2
  Delta_C/1 -> Add/1
  Lmbada_C/1 -> Add/2
  ks/1 -> Add1/2
  x_def/1 -> ks/1
  Constant1/1 -> Switch/1
  Product1/1 -> Gain/1
  Add/1 -> Product1/2
  Gain/1 -> Add1/1
  Constant/1 -> Switch/3
  v_def/1 -> Product1/1, Product/1
  Switch/1 -> Delta_C/1
  v_s/1 -> Product/2
  Add1/1 -> Out1/1

== system RL_sus_quarter_sim/Quarter_sys/Control/Y_1/SH_ADD_new_xdef_vs/2nd_FS_adef_vs ==
  vs : Inport
  adef : Inport  Port=2
  2nd_FS : Sum  Inputs=+-
  Constant4 : Constant  Value=20000
  Constant5 : Constant  Value=400
  Constant6 : Constant  Value=1000
  MATLAB Function1 : MATLAB Function  TreatAsAtomicUnit=on
  Product : Product
  Scope : Scope  NumInputPorts=2
      settings: ActiveDisplayYMinimum=-116.16886  ActiveDisplayYMaximum=1045.51973  DataLoggingVariableName=ScopeData20
  Scope1 : Scope
      settings: ActiveDisplayYMinimum=-4.46239  ActiveDisplayYMaximum=40.1615  DataLoggingVariableName=ScopeData22
  Scope2 : Scope
      settings: ActiveDisplayYMinimum=-116.16886  ActiveDisplayYMaximum=1045.51973  DataLoggingVariableName=ScopeData23
  Scope3 : Scope
      settings: ActiveDisplayYMinimum=-101.89927  ActiveDisplayYMaximum=101.85233  DataLoggingVariableName=ScopeData24
  Square : Math  Operator=square
  Square1 : Math  Operator=square
  alpha2 : Constant  Value=2*2*pi
  FS2 : Outport
  wires:
  Square1/1 -> Product/2
  vs/1 -> Square1/1
  adef/1 -> Scope3/1, MATLAB Function1/1(au)
  Product/1 -> Scope1/1, 2nd_FS/2, Scope/2
  Constant4/1 -> MATLAB Function1/3(ks)
  Constant6/1 -> MATLAB Function1/5(cs)
  MATLAB Function1/1(y) -> Scope/1, Scope2/1, 2nd_FS/1
  2nd_FS/1 -> FS2/1
  Constant5/1 -> MATLAB Function1/4(ms)
  Square/1 -> Product/1
  alpha2/1 -> MATLAB Function1/2(alpha), Square/1

== system RL_sus_quarter_sim/Quarter_sys/Control/Y_1/SH_ADD_new_xdef_vs/ADD ==
  x_def : Inport
  v_def : Inport  Port=2
  a_s : Inport  Port=3
  Add : Sum
  Add1 : Sum
  Constant7 : Constant  Value=-1
  Constant8 : Constant
  Delta_C : Gain  Gain=500
  Gain : Gain  Gain=-1
  Lmbada_C : Constant  Value=1000
  Product : Product
  Product1 : Product
  Switch : Switch  Criteria=u2 > Threshold  SaturateOnIntegerOverflow=off  InputSameDT=off
  ks : Gain  Gain=-20000
  F_sus1 : Outport
  wires:
  ks/1 -> Add1/2
  v_def/1 -> Product1/1, Product/1
  a_s/1 -> Product/2
  Constant7/1 -> Switch/3
  Switch/1 -> Delta_C/1
  Product1/1 -> Gain/1
  Product/1 -> Switch/2
  Lmbada_C/1 -> Add/2
  x_def/1 -> ks/1
  Add1/1 -> F_sus1/1
  Add/1 -> Product1/2
  Constant8/1 -> Switch/1
  Delta_C/1 -> Add/1
  Gain/1 -> Add1/1

== system RL_sus_quarter_sim/Quarter_sys/Control/Y_1/SH_ADD_new_xdef_vs/SH ==
  v_def : Inport
  v_s : Inport  Port=2
  x_def : Inport  Port=3
  Add : Sum
  Add1 : Sum
  Constant : Constant  Value=-1
  Constant1 : Constant
  Delta_C : Gain  Gain=500
  Gain : Gain  Gain=-1
  Lmbada_C : Constant  Value=1000
  Product : Product
  Product1 : Product
  Switch : Switch  Criteria=u2 > Threshold  SaturateOnIntegerOverflow=off  InputSameDT=off
  ks : Gain  Gain=-20000
  Out1 : Outport
  wires:
  Add1/1 -> Out1/1
  v_s/1 -> Product/2
  Switch/1 -> Delta_C/1
  v_def/1 -> Product/1, Product1/1
  Constant/1 -> Switch/3
  Gain/1 -> Add1/1
  Add/1 -> Product1/2
  Product1/1 -> Gain/1
  Constant1/1 -> Switch/1
  x_def/1 -> ks/1
  ks/1 -> Add1/2
  Lmbada_C/1 -> Add/2
  Delta_C/1 -> Add/1
  Product/1 -> Switch/2

== system RL_sus_quarter_sim/Quarter_sys/Control/Y_1/decouple_simple/passive ==
  In1 : Inport
  In2 : Inport  Port=2
  Add2 : Sum
  cs : Gain  Gain=-1000
  ks : Gain  Gain=-20000
  passive : Outport
  wires:
  In1/1 -> ks/1
  cs/1 -> Add2/2
  In2/1 -> cs/1
  ks/1 -> Add2/1
  Add2/1 -> passive/1  "passive"

== system RL_sus_quarter_sim/Quarter_sys/Control/Y_1/freq semi/ADD ==
  x_def : Inport
  v_def : Inport  Port=2
  a_s : Inport  Port=3
  Add : Sum
  Add1 : Sum
  Constant7 : Constant  Value=-1
  Constant8 : Constant
  Delta_C : Gain  Gain=500
  Gain : Gain  Gain=-1
  Lmbada_C : Constant  Value=1000
  Product : Product
  Product1 : Product
  Switch : Switch  Criteria=u2 > Threshold  SaturateOnIntegerOverflow=off  InputSameDT=off
  ks : Gain  Gain=-20000
  F_sus1 : Outport
  wires:
  Gain/1 -> Add1/1
  Delta_C/1 -> Add/1
  Constant8/1 -> Switch/1
  Add/1 -> Product1/2
  Add1/1 -> F_sus1/1
  x_def/1 -> ks/1
  Lmbada_C/1 -> Add/2
  Product/1 -> Switch/2
  Product1/1 -> Gain/1
  Switch/1 -> Delta_C/1
  Constant7/1 -> Switch/3
  a_s/1 -> Product/2
  v_def/1 -> Product/1, Product1/1
  ks/1 -> Add1/2

== system RL_sus_quarter_sim/Quarter_sys/Control/Y_1/freq semi/SH ==
  v_def : Inport
  v_s : Inport  Port=2
  x_def : Inport  Port=3
  Add : Sum
  Add1 : Sum
  Constant : Constant  Value=-1
  Constant1 : Constant
  Delta_C : Gain  Gain=500
  Gain : Gain  Gain=-1
  Lmbada_C : Constant  Value=1000
  Product : Product
  Product1 : Product
  Switch : Switch  Criteria=u2 > Threshold  SaturateOnIntegerOverflow=off  InputSameDT=off
  ks : Gain  Gain=-20000
  Out1 : Outport
  wires:
  Product/1 -> Switch/2
  Delta_C/1 -> Add/1
  Lmbada_C/1 -> Add/2
  ks/1 -> Add1/2
  x_def/1 -> ks/1
  Constant1/1 -> Switch/1
  Product1/1 -> Gain/1
  Add/1 -> Product1/2
  Gain/1 -> Add1/1
  Constant/1 -> Switch/3
  v_def/1 -> Product1/1, Product/1
  Switch/1 -> Delta_C/1
  v_s/1 -> Product/2
  Add1/1 -> Out1/1

== system RL_sus_quarter_sim/Quarter_sys/Control/Y_1/freq semi/Subsystem ==
  vs : Inport
  au : Inport  Port=2
  as : Inport  Port=3
  1st_FS1 : MATLAB Function  TreatAsAtomicUnit=on
  2nd_FS : Subsystem
  2nd_FS1 : Subsystem  Commented=on
  Chart : Stateflow chart  TreatAsAtomicUnit=on
  alpha2 : Constant  Value=1.5*2*pi
  Select : Outport
  FS_1 : Outport  Port=2
  FS_2 : Outport  Port=3
  wires:
  vs/1 -> 1st_FS1/2(vs), 2nd_FS1/1(vs), 2nd_FS/1(vs)
  1st_FS1/1(y) -> FS_1/1, Chart/1(FS_1)
  au/1 -> 2nd_FS1/2(au), 2nd_FS/2(au)
  2nd_FS/1(FS2) -> FS_2/1, Chart/2(FS_2)
  Chart/1(Select) -> Select/1
  as/1 -> 1st_FS1/1(as)
  alpha2/1 -> 1st_FS1/3(alpha1)

== system RL_sus_quarter_sim/Quarter_sys/Control/Y_1/freq semi/Subsystem1 ==
  v_def : Inport
  x_def : Inport  Port=2
  Add1 : Sum
  Gain : Gain  Gain=-1
  Lmbada_C : Constant  Value=1000
  Product1 : Product
  ks : Gain  Gain=-20000
  Out1 : Outport
  wires:
  Add1/1 -> Out1/1
  v_def/1 -> Product1/1
  Gain/1 -> Add1/1
  Lmbada_C/1 -> Product1/2
  Product1/1 -> Gain/1
  x_def/1 -> ks/1
  ks/1 -> Add1/2
